simulink model "DroneNonLinearModel"  (R2022b)
settings: Solver=VariableStepAuto  StartTime=0.0  StopTime=10.0  RelTol=1e-3
values from neighbouring files (symbols this model uses):
  X0 = zeros(12,1)    [DroneDynamicModel.m]    (also in Params.mat = [0 0 0 0 0 0 0 0 0 0 0 0])
undefined symbols (not defined in the file or in its folder): DroneDynamicModel
settings Model: Creator=bendr  LastModifiedBy=bendr
settings DataIOCC: ExternalInput=getinputstruct(op_trim1)  InitialState=getstatestruct(op_trim1)  LoadExternalInput=on  LoadInitialState=on

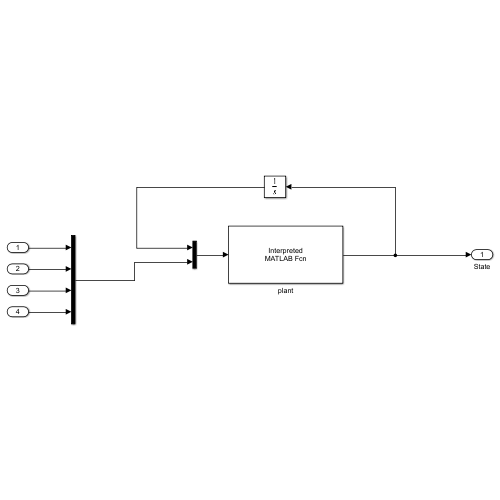
[thumbnail: Simulink's stored preview of the top-level diagram]
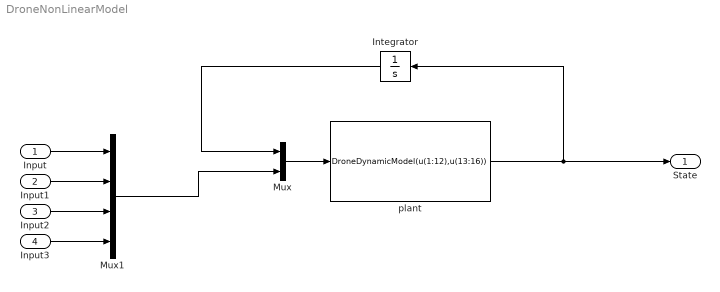
== system DroneNonLinearModel ==
  Input : Inport
  Input1 : Inport  Port=2
  Input2 : Inport  Port=3
  Input3 : Inport  Port=4
  Integrator : Integrator  InitialCondition=X0
  Mux : Mux  Inputs=2
  Mux1 : Mux
  plant : MATLABFcn  MATLABFcn=DroneDynamicModel(u(1:12),u(13:16))
  State : Outport
  wires:
  plant/1 -> Integrator/1, State/1
  Mux/1 -> plant/1
  Integrator/1 -> Mux/1
  Mux1/1 -> Mux/2
  Input/1 -> Mux1/1
  Input1/1 -> Mux1/2
  Input2/1 -> Mux1/3
  Input3/1 -> Mux1/4
